simulink model "DrivingPatternBasic_test_harness"  (R2020b)
settings: Solver=daessc  StartTime=0.0  StopTime=t_end  RelTol=1e-3  AbsTol=1e-3
PreLoadFcn:
  | DrivingPatternBasic_setup
libraries: simulink x7
settings Model: Creator=ihctr  LastModifiedBy=isaacito
settings SolverCC: AutoScaleAbsTol=off
settings DataIOCC: DSMLogging=off

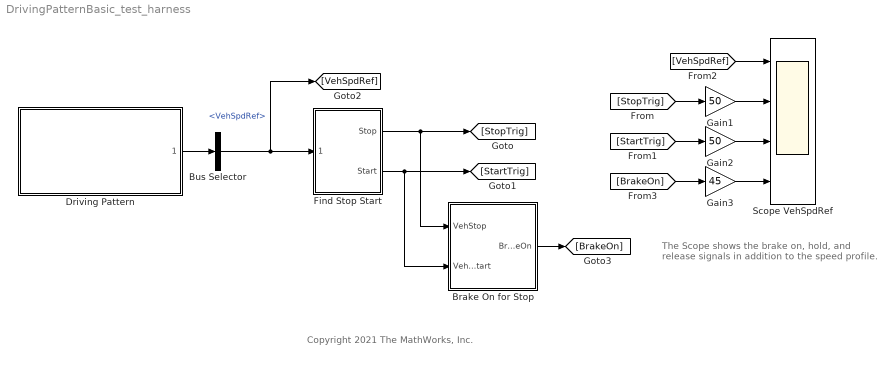
== system DrivingPatternBasic_test_harness ==
  note: The Scope shows the brake on,
      | hold, and release signals
      | in addition to the speed profile.
  note: Copyright 2021 The MathWorks, Inc.
  Brake On for Stop : Stateflow chart  TreatAsAtomicUnit=on
  Bus Selector : BusSelector  OutputSignals=VehSpdRef
  Driving Pattern : Subsystem  ReferencedSubsystem=DrivingPatternBasic_refsub
  Find Stop Start : Subsystem
  Gain1 : Gain  Gain=50
  Gain2 : Gain  Gain=50
  Gain3 : Gain  Gain=45
  Scope VehSpdRef : Scope  NumInputPorts=4
  wires:
  [StopTrig] -> Gain1/1
  Gain1/1 -> Scope VehSpdRef/2
  [StartTrig] -> Gain2/1
  Gain2/1 -> Scope VehSpdRef/3
  [VehSpdRef] -> Scope VehSpdRef/1
  [BrakeOn] -> Gain3/1
  Driving Pattern/1 -> Bus Selector/1
  Brake On for Stop/1(BrakeOn) -> [BrakeOn]
  Find Stop Start/2(Start) -> [StartTrig], Brake On for Stop/2(VehStart)
  Find Stop Start/1(Stop) -> [StopTrig], Brake On for Stop/1(VehStop)
  Bus Selector/1 -> Find Stop Start/1(VehSpd), [VehSpdRef]  "<VehSpdRef>"
  Gain3/1 -> Scope VehSpdRef/4

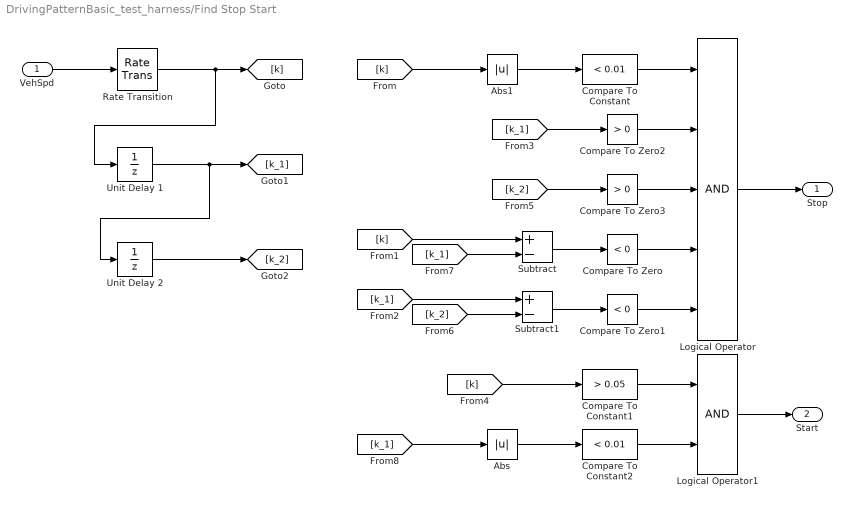
== system DrivingPatternBasic_test_harness/Find Stop Start ==
  VehSpd : Inport
  Abs : Abs
  Abs1 : Abs
  Compare To Constant : simulink/Logic and Bit Operations/Compare To Constant  relop=<  const=0.01  OutDataTypeStr=boolean
  Compare To Constant1 : simulink/Logic and Bit Operations/Compare To Constant  relop=>  const=0.05  OutDataTypeStr=boolean
  Compare To Constant2 : simulink/Logic and Bit Operations/Compare To Constant  relop=<  const=0.01  OutDataTypeStr=boolean
  Compare To Zero : simulink/Logic and Bit Operations/Compare To Zero  relop=<  OutDataTypeStr=boolean
  Compare To Zero1 : simulink/Logic and Bit Operations/Compare To Zero  relop=<  OutDataTypeStr=boolean
  Compare To Zero2 : simulink/Logic and Bit Operations/Compare To Zero  relop=>  OutDataTypeStr=boolean
  Compare To Zero3 : simulink/Logic and Bit Operations/Compare To Zero  relop=>  OutDataTypeStr=boolean
  Logical Operator : Logic  Inputs=5  AllPortsSameDT=off  OutDataTypeStr=boolean
  Logical Operator1 : Logic  AllPortsSameDT=off  OutDataTypeStr=boolean
  Rate Transition : RateTransition  OutPortSampleTime=1
      settings: AttributesFormatString=Sample Time: %<OutPortSampleTime>
  Subtract : Sum  Inputs=+-
  Subtract1 : Sum  Inputs=+-
  Unit Delay 1 : UnitDelay  HasFrameUpgradeWarning=on
      settings: AttributesFormatString=Sample Time: %<SampleTime>
  Unit Delay 2 : UnitDelay  HasFrameUpgradeWarning=on
      settings: AttributesFormatString=Sample Time: %<SampleTime>
  Stop : Outport  OutDataTypeStr=boolean
  Start : Outport  Port=2  OutDataTypeStr=boolean
  wires:
  Rate Transition/1 -> Unit Delay 1/1, [k]
  Subtract/1 -> Compare To Zero/1
  Subtract1/1 -> Compare To Zero1/1
  Compare To Constant/1 -> Logical Operator/1
  Compare To Zero2/1 -> Logical Operator/2
  Compare To Zero1/1 -> Logical Operator/5
  Logical Operator/1 -> Stop/1
  [k] -> Abs1/1
  [k] -> Subtract/1
  [k_1] -> Subtract1/1
  Unit Delay 1/1 -> Unit Delay 2/1, [k_1]
  [k_1] -> Compare To Zero2/1
  Unit Delay 2/1 -> [k_2]
  [k_2] -> Compare To Zero3/1
  [k_2] -> Subtract1/2
  [k_1] -> Subtract/2
  Compare To Zero3/1 -> Logical Operator/3
  Compare To Zero/1 -> Logical Operator/4
  Compare To Constant1/1 -> Logical Operator1/1
  [k] -> Compare To Constant1/1
  [k_1] -> Abs/1
  Compare To Constant2/1 -> Logical Operator1/2
  Logical Operator1/1 -> Start/1
  Abs/1 -> Compare To Constant2/1
  Abs1/1 -> Compare To Constant/1
  VehSpd/1 -> Rate Transition/1

== stateflow chart DrivingPatternBasic_test_harness/Brake On for Stop ==
  state BrakeOn
    entry:
    BrakeOn = true;
  state Initial
  state BrakeOff
    entry:
    BrakeOn = false;
  (junction 10) -> BrakeOn : [VehStop == true]
  Initial -> (junction 10) [order 1]
  BrakeOff -> BrakeOn : [VehStop == true]
  BrakeOn -> BrakeOff : [VehStart == true]
  (default) -> Initial
  Initial -> (junction 12) [order 2]
  (junction 12) -> BrakeOff : [VehStart == true]
  data: VehStop input; BrakeOn output; VehStart input
